simulink model "CCCS_lin_in_comm_out_comm"  (Simulink 7.5)
settings: Solver=ode45  StartTime=0.0  StopTime=10.0  RelTol=1e-3
settings Model: Creator=tugui_cat  LastModifiedBy=tugui
settings DebuggingCC: StrictBusMsg=Warning

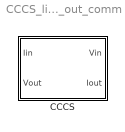
== system CCCS_lin_in_comm_out_comm ==
  CCCS : Subsystem  mask{Num_TF_dir1=1, Den_TF_dir1=1, Num_TF_inv1=1, Den_TF_inv1=1, Num_Zin1=1, Den_Zin1=1, Num_Zout1=1, Den_Zout1=1, OffIn11=0, OffIn12=0, OffOut11=0, OffOut12=0}
      mask help: Current-Controlled-Current-Source - linear model

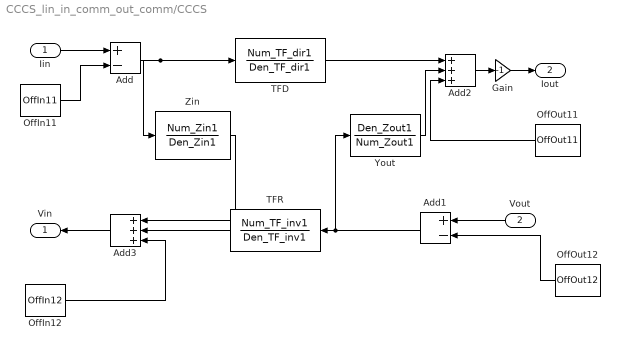
== system CCCS_lin_in_comm_out_comm/CCCS ==
  Iin : Inport
  Vout : Inport  Port=2
  Add : Sum  Inputs=+-  OutDataType=fixdt(1, 16)  OutScaling=2^-10
  Add1 : Sum  Inputs=+-  OutDataType=fixdt(1, 16)  OutScaling=2^-10
  Add2 : Sum  Inputs=+++  OutDataType=fixdt(1, 16)  OutScaling=2^-10
  Add3 : Sum  Inputs=+++  OutDataType=fixdt(1, 16)  OutScaling=2^-10
  Gain : Gain  Gain=-1  ParameterDataType=fixdt(1, 16)  ParameterScaling=2^0  OutDataType=fixdt(1, 16)  OutScaling=2^0
  OffIn11 : Constant  Value=OffIn11  OutDataType=fixdt(1, 16)  OutScaling=2^0
  OffIn12 : Constant  Value=OffIn12  OutDataType=fixdt(1, 16)  OutScaling=2^0
  OffOut11 : Constant  Value=OffOut11  OutDataType=fixdt(1, 16)  OutScaling=2^0
  OffOut12 : Constant  Value=OffOut12  OutDataType=fixdt(1, 16)  OutScaling=2^0
  TFD : TransferFcn  Numerator=Num_TF_dir1  Denominator=Den_TF_dir1
  TFR : TransferFcn  Numerator=Num_TF_inv1  Denominator=Den_TF_inv1
  Yout : TransferFcn  Numerator=Den_Zout1  Denominator=Num_Zout1
  Zin : TransferFcn  Numerator=Num_Zin1  Denominator=Den_Zin1
  Vin : Outport
  Iout : Outport  Port=2
  wires:
  TFD/1 -> Add2/1
  Add3/1 -> Vin/1
  Zin/1 -> Add3/1
  TFR/1 -> Add3/2
  Yout/1 -> Add2/2
  Iin/1 -> Add/1
  Add/1 -> Zin/1, TFD/1
  OffIn11/1 -> Add/2
  Vout/1 -> Add1/1
  Add1/1 -> Yout/1, TFR/1
  OffOut12/1 -> Add1/2
  OffOut11/1 -> Add2/3
  OffIn12/1 -> Add3/3
  Add2/1 -> Gain/1
  Gain/1 -> Iout/1
